simulink model "purepursuitcontrol"  (R2021a)
settings: Solver=VariableStepAuto  StartTime=0.0  StopTime=sim_time  RelTol=1e-3
values from neighbouring files (symbols this model uses):
  L = 4.7    [purepursuitcontroller.m]
  Ld = 10    [purepursuitcontroller.m]
  psi_0 = 0    [purepursuitcontroller.m]
  Vref = 30    [purepursuitcontroller.m]
  X_0 = xRef(1,1)    [purepursuitcontroller.m]
  xRef = refPose(1,:)    [purepursuitcontroller.m]
  Y_0 = yRef(1,1)    [purepursuitcontroller.m]
  yRef = refPose(2,:)    [purepursuitcontroller.m]
libraries: autolibshared x1, robotalgslib x1
settings Model: Creator=User  LastModifiedBy=User

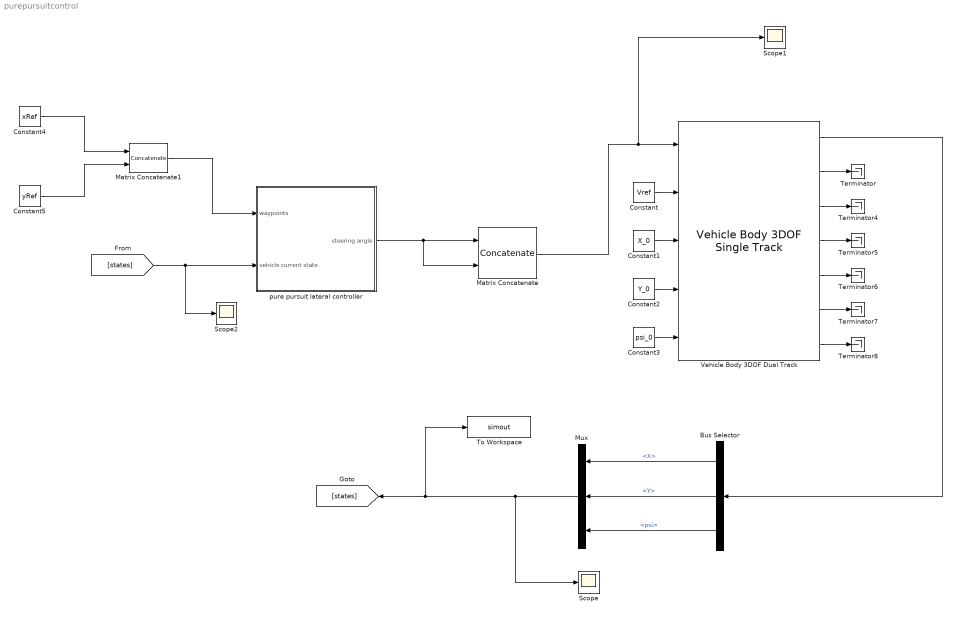
== system purepursuitcontrol ==
  Bus Selector : BusSelector  OutputSignals=InertFrm.Cg.Disp.X,InertFrm.Cg.Disp.Y,InertFrm.Cg.Ang.psi
  Constant : Constant  Value=Vref
  Constant1 : Constant  Value=X_0
  Constant2 : Constant  Value=Y_0
  Constant3 : Constant  Value=psi_0
  Constant4 : Constant  Value=xRef
  Constant5 : Constant  Value=yRef
  Matrix Concatenate : Concatenate  ConcatenateDimension=2
  Matrix Concatenate1 : Concatenate  Mode=Multidimensional array  ConcatenateDimension=2
  Mux : Mux  Inputs=3
  Scope : Scope
  Scope1 : Scope
  Scope2 : Scope
  Terminator{,4..8} (6 alike) : Terminator
  To Workspace : ToWorkspace  VariableName=simout  SaveFormat=Timeseries  SampleTime=-1
  Vehicle Body 3DOF Dual Track : autolibshared/Vehicle Body 3DOF Single Track  trackMode=Dual  inputMode=External longitudinal velocity  frontSteerMode=on  rearSteerMode=off  windMode=off  muMode=off  extFMode=off  extMMode=off  htchFMode=off  htchMMode=off  extXo=on  extpsio=on  extxdoto=off  extro=off  extYo=on  extTamb=off  extydoto=off  aMode=2  NF=2  NR=2  m=2000  a=1.4  b=1.6  h=0.35  dh=1  hh=0.2  X_o=0  xdot_o=0  CalphaMode=off  sigmaMode=on  d=0  hl=0  w=[1.4,1.4]  Cy_f=12e3  Cy_r=11e3  sigma_f=.1  sigma_r=.1  alpha_f_brk=[-.1 .1]  Cy_f_data=[-9e3 9e3]  alpha_r_brk=[-.1 .1]  Cy_r_data=[-9e3 9e3]  Y_o=0  ydot_o=0  Izz=4000  psi_o=0  r_o=0  Af=2  Cd=.3  Cl=.1  Cpm=.1  beta_w=[0:0.01:0.3]  Cs=[0:0.03:0.9]  Cym=[0:0.01:0.3]  Pabs=101325  Tair=273  g=9.81  mu=1  xdot_tol=.01  Fznom=5000  Fxtire_sat=7e4  Fytire_sat=7e4  longOff=0  latOff=0  vertOff=0  wrapAng=off
      settings: SourceProductBaseCode=PW,DR,MT,UV,VE
  pure pursuit lateral controller : Subsystem
  wires:
  pure pursuit lateral controller/1(steering angle) -> Matrix Concatenate/2, Matrix Concatenate/1
  Matrix Concatenate/1 -> Scope1/1, Vehicle Body 3DOF Dual Track/1
  Constant/1 -> Vehicle Body 3DOF Dual Track/2
  Constant1/1 -> Vehicle Body 3DOF Dual Track/3
  Constant2/1 -> Vehicle Body 3DOF Dual Track/4
  Constant3/1 -> Vehicle Body 3DOF Dual Track/5
  Vehicle Body 3DOF Dual Track/2 -> Terminator/1
  Vehicle Body 3DOF Dual Track/3 -> Terminator4/1
  Vehicle Body 3DOF Dual Track/4 -> Terminator5/1
  Vehicle Body 3DOF Dual Track/5 -> Terminator6/1
  Vehicle Body 3DOF Dual Track/6 -> Terminator7/1
  Vehicle Body 3DOF Dual Track/7 -> Terminator8/1
  Vehicle Body 3DOF Dual Track/1 -> Bus Selector/1
  Bus Selector/1 -> Mux/1  "<X>"
  Bus Selector/2 -> Mux/2  "<Y>"
  Bus Selector/3 -> Mux/3  "<psi>"
  Mux/1 -> Scope/1, To Workspace/1, [states]
  [states] -> Scope2/1, pure pursuit lateral controller/2(vehicle current state)
  Constant4/1 -> Matrix Concatenate1/1
  Constant5/1 -> Matrix Concatenate1/2
  Matrix Concatenate1/1 -> pure pursuit lateral controller/1(waypoints)

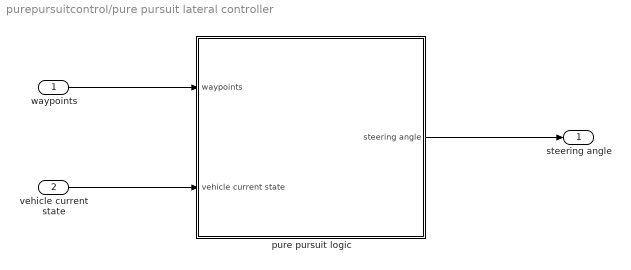
== system purepursuitcontrol/pure pursuit lateral controller ==
  waypoints : Inport
  vehicle current state : Inport  Port=2
  pure pursuit logic : Subsystem
  steering angle : Outport
  wires:
  waypoints/1 -> pure pursuit logic/1(waypoints)
  vehicle current state/1 -> pure pursuit logic/2(vehicle current state)
  pure pursuit logic/1(steering angle) -> steering angle/1

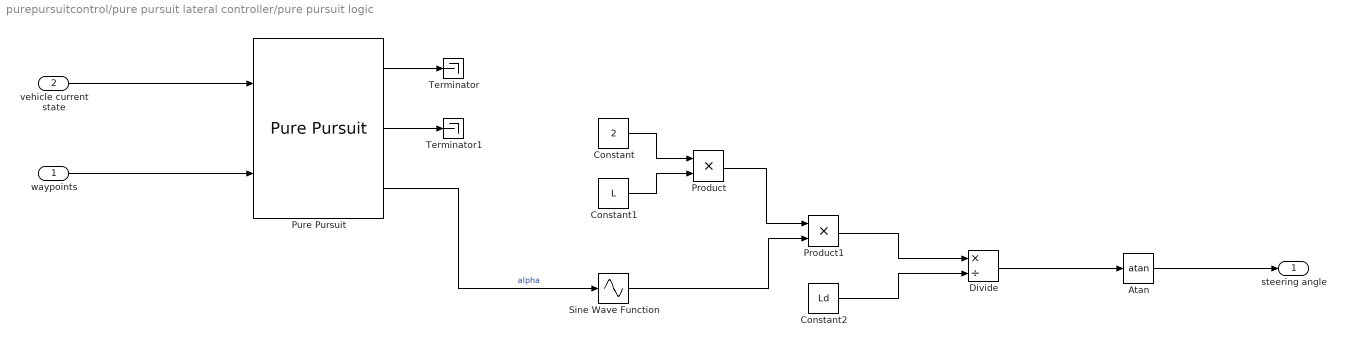
== system purepursuitcontrol/pure pursuit lateral controller/pure pursuit logic ==
  waypoints : Inport
  vehicle current state : Inport  Port=2
  Atan : Trigonometry  Operator=atan
  Constant : Constant  Value=2
  Constant1 : Constant  Value=L
  Constant2 : Constant  Value=Ld
  Divide : Product  Inputs=*/
  Product : Product
  Product1 : Product
  Pure Pursuit : robotalgslib/Pure Pursuit  DesiredLinearVelocity=Vref  MaxAngularVelocity=1.0  LookaheadDistance=Ld  TargetDirPort=on  SimulateUsing=Code generation
  Sine Wave Function : Sin  TimeSource=Use external signal  SampleTime=0
  Terminator : Terminator
  Terminator1 : Terminator
  steering angle : Outport
  wires:
  vehicle current state/1 -> Pure Pursuit/1
  waypoints/1 -> Pure Pursuit/2
  Pure Pursuit/1 -> Terminator/1
  Pure Pursuit/2 -> Terminator1/1
  Pure Pursuit/3 -> Sine Wave Function/1  "alpha"
  Constant/1 -> Product/1
  Constant1/1 -> Product/2
  Product/1 -> Product1/1
  Sine Wave Function/1 -> Product1/2
  Product1/1 -> Divide/1
  Constant2/1 -> Divide/2
  Divide/1 -> Atan/1
  Atan/1 -> steering angle/1
